simulink model "aabb"  (R2020b)
settings: Solver=VariableStepAuto  StartTime=0.0  StopTime=0.2  MaxStep=1/400  RelTol=1e-3
settings Model: Creator=seojoon  LastModifiedBy=seojoon

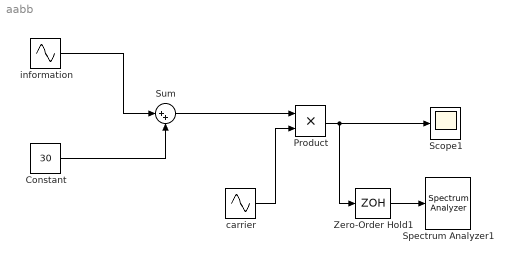
== system aabb ==
  Constant : Constant  Value=30
  Product : Product
  Scope1 : Scope
  Spectrum Analyzer1 : SpectrumAnalyzer
  Sum : Sum  Inputs=|++
  Zero-Order Hold1 : ZeroOrderHold  SampleTime=1/20000
  carrier : Sin  Amplitude=30  Frequency=2*pi*1000  Phase=pi/2  SampleTime=0
  information : Sin  Amplitude=0.3  Frequency=2*pi*3000  SampleTime=0
  wires:
  information/1 -> Sum/1
  Constant/1 -> Sum/2
  Sum/1 -> Product/1
  carrier/1 -> Product/2
  Product/1 -> Zero-Order Hold1/1, Scope1/1
  Zero-Order Hold1/1 -> Spectrum Analyzer1/1
